simulink model "VIRTUAL_self_driving_stack_v2"  (R2025b)
settings: Solver=ode1  StartTime=0.0  StopTime=inf  FixedStep=Controller_Sample_Time  RelTol=1e-3  EnableMultiTasking=on
values from neighbouring files (symbols this model uses):
  angles_qcar2 = angles_new_qcar2(2: length (angles_new_qcar2), width (angles_new_qcar2)-5)    [Setup_QCar2_Params.m]
  cal_pos = [0, 0, 0]    [Setup_QCar2_Params.m]
  Controller_Sample_Time = 1/500    (= 0.002)    [Setup_QCar2_Params.m]
  CSI_Sample_Time = Controller_Sample_Time * ceil(0.033 / Controller_Sample_Time)    [Setup_QCar2_Params.m]
  dropoffXY = pathXY(dropoffPathIndex,:)    [example_sdcs_path.m]
  GyroKF_P0 = eye(2)    [Setup_QCar2_Params.m]
  GyroKF_Q = diag([0.01, 0.001])    [Setup_QCar2_Params.m]
  GyroKF_R = 0.01    [Setup_QCar2_Params.m]
  GyroKF_X0 = [0;0]    [Setup_QCar2_Params.m]
  ImageDisplay_Sample_Time = Controller_Sample_Time * 50    (= 0.1)    [Setup_QCar2_Params.m]
  Initialization_Time = 5    [Setup_QCar2_Params.m]
  LiDAR_Sample_Time = Controller_Sample_Time * ceil(1/15 / Controller_Sample_Time)    [Setup_QCar2_Params.m]
  N = size(roadmap.nodes,1)    [example_sdcs_path.m]
  path_x4 = path_x_custom    [Setup_QCar2_Params.m]
  path_y4 = path_y_custom    [Setup_QCar2_Params.m]
  pickupXY = pathXY(pickupPathIndex,:)    [example_sdcs_path.m]
  qcar2_lidar_to_body_rotation = -pi    (= -3.14159265359)    [Setup_QCar2_Params.m]
  qcar2_lidar_to_map_rotation = 2*pi/180    (= 0.0349065850399)    [Setup_QCar2_Params.m]
  qcar2_virtual_to_physical_lidar_rotation = 0    [Setup_QCar2_Params.m]
  QCarEKF_L = 0.256    [Setup_QCar2_Params.m]
  QCarEKF_P0 = eye(3)    [Setup_QCar2_Params.m]
  QCarEKF_Q = diag([0.00001, 0.00001, 0.00001])    [Setup_QCar2_Params.m]
  QCarEKF_R_combined = diag([0.1, 0.1, 0.01])    [Setup_QCar2_Params.m]
  QCarEKF_R_heading = diag(0.1)    [Setup_QCar2_Params.m]
  QcarKF_X0 = [0; 0; 0]    [Setup_QCar2_Params.m]
  range_qcar2 = distance_new_qcar2(2: length (distance_new_qcar2), width (distance_new_qcar2)-5)    [Setup_QCar2_Params.m]
  RealSense_Sample_Time = Controller_Sample_Time * ceil(0.033 / Controller_Sample_Time)    [Setup_QCar2_Params.m]
  steering_Kd = 0.1    [Setup_QCar2_Params.m]
  taxiHubXY = pathXY(taxiHubPathIndex,:)    [example_sdcs_path.m]
  x = roadmap.nodes(i,1)    [example_sdcs_path.m]
undefined symbols (not defined in the file or in its folder): AAAF5050, gcbh, height, HIL, JPEG, K12, left, MC, Point, qc_get_step_size, top, Video3D, video_display_show, width
libraries: quarc_library x76, simulink x17, simulink_extras x4, visiontextngfix x1
(part 4 of 4)

== system VIRTUAL_self_driving_stack_v2/Image Processing/ImageProcessingBlock/colorThresholdingHSV ==
  note: Generate the thresholded binary
  note: Transform RGB Image to an HSV one
  note: Color wheel
      | reference
      | for Hue_360
  note: HSV-Color Thresholding Module:
      |
      | This subsystem thresholds a given RGB image based on the desired colour and hue
      |
      | Inputs:
      | imageRGB (uint8) {0,255} : Input RGB Image to be thresholded
      | desiredHue (int) {-1}U{0,360} : Desired Hue to threshold around (provided in the 0-360 degree range, see the color wheel for hue selection)
      | Set the desired hue to -1 if you are interested in thresholding for white
      | [Sat_min, Val_min] (uint8) {0,255} : Minimum Saturation and Value thresholds
      | [Sat_max, Val_max] (uint8) {0,255} : Maximum Saturation and Value thresholds
      |
      | Outputs:
      | imageBinary (uint8) {0,255} : Binary Image (0 or 255 and no other value) representing the thresholding output
      |
      | Usage:
      | This module can be used when you are interested in thresholding for a certain hue regardless of the luminance. Compared to RGB thresholding which does not work well when the lighting conditions vary, HSV thresholding will correctly threshold for a hue (color) and allow you to specify a broad range of illuminance via the saturation and value thresholds. To broaden the range of hues accepted in the thresholding block, increase the Hue Threshold parameter.
  imageHSV : Inport
  desiredHue : Inport  Port=2
  "[Sat_min, Val_min]" : Inport  Port=3
  "[Sat_max, Val_max]" : Inport  Port=4
  Add3 : Sum
  Add4 : Sum  Inputs=-+
  Compare To Constant : simulink/Logic and Bit Operations/Compare To Constant  relop===  const=-1  OutDataTypeStr=boolean
  Constant : Constant  Value=0
  Constant1 : Constant  Value=255
  Display : Display
  Gain : Gain  Gain=255/360
  HSV Color Thresholding : quarc_library/Image Processing/Generic/Image Compare  output_type=Combined (one HxW output)  source=External input ports  r_comparison=min <= pixel and pixel <= max with wrapping  r_minimum=30  r_maximum=70  g_comparison=min <= pixel and pixel <= max  g_minimum=60  g_maximum=100  b_comparison=min <= pixel and pixel <= max  b_minimum=40  b_maximum=80
      settings: SourceProductName=QUARC Targets
  Hue Threshold : Constant  Value=20
  Mux1 : Mux  Inputs=2
  Mux2 : Mux  Inputs=2
  Switch : Switch  Criteria=u2 > Threshold  SaturateOnIntegerOverflow=off  InputSameDT=off
  Switch1 : Switch  Criteria=u2 > Threshold  SaturateOnIntegerOverflow=off  InputSameDT=off
  imageBinary : Outport  VectorParamsAs1DForOutWhenUnconnected=off
  wires:
  Hue Threshold/1 -> Add3/1, Add4/1
  imageHSV/1 -> HSV Color Thresholding/1
  desiredHue/1 -> Compare To Constant/1, Display/1, Gain/1
  Gain/1 -> Add4/2, Add3/2
  Constant1/1 -> Switch1/1
  "[Sat_max, Val_max]"/1 -> Mux1/2
  Add3/1 -> Switch1/3
  Switch/1 -> Mux2/1
  Compare To Constant/1 -> Switch/2, Switch1/2
  Constant/1 -> Switch/1
  Switch1/1 -> Mux1/1
  Mux1/1 -> HSV Color Thresholding/3
  Add4/1 -> Switch/3
  "[Sat_min, Val_min]"/1 -> Mux2/2
  Mux2/1 -> HSV Color Thresholding/2
  HSV Color Thresholding/1 -> imageBinary/1

== system VIRTUAL_self_driving_stack_v2/Image Processing/findStopSignDistance/Depth Image (m) ==
  In1 : Inport
  Channel : quarc_library/Signal Routing/Channel  channel=5  buffer_size=1
  Image Compress : quarc_library/Image Processing/Generic/Image Compress  algorithm=JPEG  source=Internal dialog parameter  quality=quality  output_dim=-1
  Video Display : quarc_library/Multimedia/Video Display  Tag=VIRTUAL_self_driving_stack_v2/Image Processing/findStopSignDistance/Depth Image (m)/Video Display  sample_time=sample_time  use_hardware=on
  wires:
  Image Compress/1 -> Channel/1
  In1/1 -> Image Compress/1
  Channel/1 -> Video Display/1

== system VIRTUAL_self_driving_stack_v2/lidarLocalization/rising edge latch/Latch Input ==
  Input : Inport
  Trigger : TriggerPort  VariantControl=(inherit)
  Constant : Constant
  Latch : Outport  VectorParamsAs1DForOutWhenUnconnected=off
  Executed : Outport  Port=2  VectorParamsAs1DForOutWhenUnconnected=off
  wires:
  Constant/1 -> Executed/1
  Input/1 -> Latch/1

== system VIRTUAL_self_driving_stack_v2/stateEstimation/Fusion Comparison & Kalman Estimator/Angle mod1 ==
  Angle : Inport
  Bias : Bias  Bias=180  SaturateOnIntegerOverflow=off
  Bias1 : Bias  Bias=-180  SaturateOnIntegerOverflow=off
  Constant1 : Constant  Value=360
  Mod : Math  Operator=mod
  Mod_Angle : Outport
  wires:
  Angle/1 -> Bias/1
  Bias1/1 -> Mod_Angle/1
  Bias/1 -> Mod/1
  Constant1/1 -> Mod/2
  Mod/1 -> Bias1/1

== system VIRTUAL_self_driving_stack_v2/steeringCommander/Steering Based on LiDAR/If Action Subsystem ==
  aoa [1] (rad) : Inport
  Action Port : ActionPort  ActionPortLabel=if(u1 < -pi)
  Bias : Bias  Bias=2*pi  SaturateOnIntegerOverflow=off
  steering [1] (rad) : Outport
  wires:
  aoa [1] (rad)/1 -> Bias/1
  Bias/1 -> steering [1] (rad)/1

== system VIRTUAL_self_driving_stack_v2/steeringCommander/Steering Based on LiDAR/If Action Subsystem1 ==
  aoa [1] (rad) : Inport
  Action Port : ActionPort  ActionPortLabel=elseif(u1 > pi)
  Bias : Bias  Bias=-2*pi  SaturateOnIntegerOverflow=off
  steering [1] (rad) : Outport
  wires:
  Bias/1 -> steering [1] (rad)/1
  aoa [1] (rad)/1 -> Bias/1

== system VIRTUAL_self_driving_stack_v2/steeringCommander/Steering Based on LiDAR/If Action Subsystem2 ==
  aoa [1] (rad) : Inport
  Action Port : ActionPort  ActionPortLabel=else
  Bias : Bias  SaturateOnIntegerOverflow=off
  steering [1] (rad) : Outport
  wires:
  aoa [1] (rad)/1 -> Bias/1
  Bias/1 -> steering [1] (rad)/1

== system VIRTUAL_self_driving_stack_v2/Image Processing/ImageProcessingBlock/DetectTrafficLight/Binary showing Green ==
  In1 : Inport
  Channel : quarc_library/Signal Routing/Channel  channel=2  buffer_size=1
  Image Compress : quarc_library/Image Processing/Generic/Image Compress  algorithm=JPEG  source=Internal dialog parameter  quality=quality  output_dim=-1
  Video Display : quarc_library/Multimedia/Video Display  Tag=VIRTUAL_self_driving_stack_v2/Image Processing/ImageProcessingBlock/DetectTrafficLight/Binary showing Green/Video Display  sample_time=sample_time  use_hardware=on
  wires:
  Image Compress/1 -> Channel/1
  In1/1 -> Image Compress/1
  Channel/1 -> Video Display/1

== system VIRTUAL_self_driving_stack_v2/Image Processing/ImageProcessingBlock/DetectTrafficLight/Binary showing Red ==
  In1 : Inport
  Channel : quarc_library/Signal Routing/Channel  channel=3  buffer_size=1
  Image Compress : quarc_library/Image Processing/Generic/Image Compress  algorithm=JPEG  source=Internal dialog parameter  quality=quality  output_dim=-1
  Video Display : quarc_library/Multimedia/Video Display  Tag=VIRTUAL_self_driving_stack_v2/Image Processing/ImageProcessingBlock/DetectTrafficLight/Binary showing Red/Video Display  sample_time=sample_time  use_hardware=on
  wires:
  Image Compress/1 -> Channel/1
  In1/1 -> Image Compress/1
  Channel/1 -> Video Display/1

== system VIRTUAL_self_driving_stack_v2/Image Processing/ImageProcessingBlock/DetectTrafficLight/colorThresholdingGreen ==
  note: Generate the thresholded binary
  note: Transform RGB Image to an HSV one
  note: Color wheel
      | reference
      | for Hue_360
  note: HSV-Color Thresholding Module:
      |
      | This subsystem thresholds a given RGB image based on the desired colour and hue
      |
      | Inputs:
      | imageRGB (uint8) {0,255} : Input RGB Image to be thresholded
      | desiredHue (int) {-1}U{0,360} : Desired Hue to threshold around (provided in the 0-360 degree range, see the color wheel for hue selection)
      | Set the desired hue to -1 if you are interested in thresholding for white
      | [Sat_min, Val_min] (uint8) {0,255} : Minimum Saturation and Value thresholds
      | [Sat_max, Val_max] (uint8) {0,255} : Maximum Saturation and Value thresholds
      |
      | Outputs:
      | imageBinary (uint8) {0,255} : Binary Image (0 or 255 and no other value) representing the thresholding output
      |
      | Usage:
      | This module can be used when you are interested in thresholding for a certain hue regardless of the luminance. Compared to RGB thresholding which does not work well when the lighting conditions vary, HSV thresholding will correctly threshold for a hue (color) and allow you to specify a broad range of illuminance via the saturation and value thresholds. To broaden the range of hues accepted in the thresholding block, increase the Hue Threshold parameter.
  imageHSV : Inport
  desiredHue : Inport  Port=2
  "[Sat_min, Val_min]" : Inport  Port=3
  "[Sat_max, Val_max]" : Inport  Port=4
  Add3 : Sum
  Add4 : Sum  Inputs=-+
  Compare To Constant : simulink/Logic and Bit Operations/Compare To Constant  relop===  const=-1  OutDataTypeStr=boolean
  Constant : Constant  Value=0
  Constant1 : Constant  Value=255
  Display : Display
  Gain : Gain  Gain=255/360
  HSV Color Thresholding : quarc_library/Image Processing/Generic/Image Compare  output_type=Combined (one HxW output)  source=External input ports  r_comparison=min <= pixel and pixel <= max with wrapping  r_minimum=30  r_maximum=70  g_comparison=min <= pixel and pixel <= max  g_minimum=60  g_maximum=100  b_comparison=min <= pixel and pixel <= max  b_minimum=40  b_maximum=80
      settings: SourceProductName=QUARC Targets
  Hue Threshold : Constant  Value=20
  Mux1 : Mux  Inputs=2
  Mux2 : Mux  Inputs=2
  Switch : Switch  Criteria=u2 > Threshold  SaturateOnIntegerOverflow=off  InputSameDT=off
  Switch1 : Switch  Criteria=u2 > Threshold  SaturateOnIntegerOverflow=off  InputSameDT=off
  imageBinary : Outport  VectorParamsAs1DForOutWhenUnconnected=off
  wires:
  Hue Threshold/1 -> Add3/1, Add4/1
  imageHSV/1 -> HSV Color Thresholding/1
  desiredHue/1 -> Compare To Constant/1, Display/1, Gain/1
  Gain/1 -> Add4/2, Add3/2
  Constant1/1 -> Switch1/1
  "[Sat_max, Val_max]"/1 -> Mux1/2
  Add3/1 -> Switch1/3
  Switch/1 -> Mux2/1
  Compare To Constant/1 -> Switch/2, Switch1/2
  Constant/1 -> Switch/1
  Switch1/1 -> Mux1/1
  Mux1/1 -> HSV Color Thresholding/3
  Add4/1 -> Switch/3
  "[Sat_min, Val_min]"/1 -> Mux2/2
  Mux2/1 -> HSV Color Thresholding/2
  HSV Color Thresholding/1 -> imageBinary/1

== system VIRTUAL_self_driving_stack_v2/Image Processing/ImageProcessingBlock/DetectTrafficLight/colorThresholdingRed ==
  note: Generate the thresholded binary
  note: Transform RGB Image to an HSV one
  note: Color wheel
      | reference
      | for Hue_360
  note: HSV-Color Thresholding Module:
      |
      | This subsystem thresholds a given RGB image based on the desired colour and hue
      |
      | Inputs:
      | imageRGB (uint8) {0,255} : Input RGB Image to be thresholded
      | desiredHue (int) {-1}U{0,360} : Desired Hue to threshold around (provided in the 0-360 degree range, see the color wheel for hue selection)
      | Set the desired hue to -1 if you are interested in thresholding for white
      | [Sat_min, Val_min] (uint8) {0,255} : Minimum Saturation and Value thresholds
      | [Sat_max, Val_max] (uint8) {0,255} : Maximum Saturation and Value thresholds
      |
      | Outputs:
      | imageBinary (uint8) {0,255} : Binary Image (0 or 255 and no other value) representing the thresholding output
      |
      | Usage:
      | This module can be used when you are interested in thresholding for a certain hue regardless of the luminance. Compared to RGB thresholding which does not work well when the lighting conditions vary, HSV thresholding will correctly threshold for a hue (color) and allow you to specify a broad range of illuminance via the saturation and value thresholds. To broaden the range of hues accepted in the thresholding block, increase the Hue Threshold parameter.
  imageHSV : Inport
  desiredHue : Inport  Port=2
  "[Sat_min, Val_min]" : Inport  Port=3
  "[Sat_max, Val_max]" : Inport  Port=4
  Add3 : Sum
  Add4 : Sum  Inputs=-+
  Compare To Constant : simulink/Logic and Bit Operations/Compare To Constant  relop===  const=-1  OutDataTypeStr=boolean
  Constant : Constant  Value=0
  Constant1 : Constant  Value=255
  Display : Display
  Gain : Gain  Gain=255/360
  HSV Color Thresholding : quarc_library/Image Processing/Generic/Image Compare  output_type=Combined (one HxW output)  source=External input ports  r_comparison=min <= pixel and pixel <= max with wrapping  r_minimum=30  r_maximum=70  g_comparison=min <= pixel and pixel <= max  g_minimum=60  g_maximum=100  b_comparison=min <= pixel and pixel <= max  b_minimum=40  b_maximum=80
      settings: SourceProductName=QUARC Targets
  Hue Threshold : Constant  Value=20
  Mux1 : Mux  Inputs=2
  Mux2 : Mux  Inputs=2
  Switch : Switch  Criteria=u2 > Threshold  SaturateOnIntegerOverflow=off  InputSameDT=off
  Switch1 : Switch  Criteria=u2 > Threshold  SaturateOnIntegerOverflow=off  InputSameDT=off
  imageBinary : Outport  VectorParamsAs1DForOutWhenUnconnected=off
  wires:
  Hue Threshold/1 -> Add3/1, Add4/1
  imageHSV/1 -> HSV Color Thresholding/1
  desiredHue/1 -> Compare To Constant/1, Display/1, Gain/1
  Gain/1 -> Add4/2, Add3/2
  Constant1/1 -> Switch1/1
  "[Sat_max, Val_max]"/1 -> Mux1/2
  Add3/1 -> Switch1/3
  Switch/1 -> Mux2/1
  Compare To Constant/1 -> Switch/2, Switch1/2
  Constant/1 -> Switch/1
  Switch1/1 -> Mux1/1
  Mux1/1 -> HSV Color Thresholding/3
  Add4/1 -> Switch/3
  "[Sat_min, Val_min]"/1 -> Mux2/2
  Mux2/1 -> HSV Color Thresholding/2
  HSV Color Thresholding/1 -> imageBinary/1

== matlab function VIRTUAL_self_driving_stack_v2/stateEstimation/Sensor Fusion - Complementary Filter/MATLAB Function ==
  data: car_speed input; correction_weight output; slope input; min_weight input
function correction_weight = weighting(car_speed, slope, min_weight)
correction_weight = 1 - 1*slope*car_speed;
if correction_weight < min_weight
    correction_weight = min_weight;
end
end

== matlab function VIRTUAL_self_driving_stack_v2/Image Processing/ImageProcessingBlock/DetectTrafficLight/MATLAB Function ==
  data: imageHSV input; meanV output; imageBinary input
function meanV = computeMeanV(imageHSV, imageBinary)
% imageHSV: HxWx3 uint8
% imageBinary: HxW uint8, values 0 or 255

V = imageHSV(:,:,3);

mask = imageBinary > 0;

vals = V(mask);

if isempty(vals)
    meanV = 0;
else
    meanV = mean(double(vals));
end

== matlab function VIRTUAL_self_driving_stack_v2/Image Processing/ImageProcessingBlock/DetectTrafficLight/MATLAB Function1 ==
  data: imageHSV input; meanV output; imageBinary input
function meanV = computeMeanV(imageHSV, imageBinary)
%#codegen
V = imageHSV(:,:,3);
mask = imageBinary > 0;
vals = V(mask);

if isempty(vals)
    meanV = 0;
else
    % If we find even ONE red pixel, return 255 to force the stop
    % This helps us check if the HSV mask is working
    meanV = 255; 
end

== matlab function VIRTUAL_self_driving_stack_v2/Image Processing/ImageProcessingBlock/MATLAB Function2 ==
  data: circularity output; box input; area input; extent output
function [circularity,extent] = detect_sign_from_area(box, area)

%#codegen
% sign_type:
% 0 = unknown
% 1 = yield
% 2 = stop


% Extract box
min_row = double(box(1));
min_col = double(box(2));
max_row = double(box(3));
max_col = double(box(4));

% Compute dimensions
height = max_row - min_row;
width  = max_col - min_col;

% Approximate perimeter
perimeter = 2 * (height + width);

% Circularity
circularity = 4 * pi * double(area) / (perimeter^2);

% Extent (how filled the box is)
box_area = height * width;
extent = double(area) / double(box_area);

% ---------- CLASSIFICATION ----------

% STOP (octagon)
% if circularity > 0.7 && extent > 0.6
%     sign_type = uint8(2);
% 
% % YIELD (triangle)
% elseif circularity > 0.45 && circularity < 0.7 && extent < 0.7
%     sign_type = uint8(1);
% 
% else
%     sign_type = uint8(0);
% end

end

== matlab function VIRTUAL_self_driving_stack_v2/speedController/realsenseObstacleDetectionSpeedAdjust/MATLAB Function ==
  data: obstacle_distance input; speed_cmd output; stop_distance input; nominal_tracking_distance input; nominal_speed input
function speed_cmd = adaptive_cruise_control(obstacle_distance, stop_distance, nominal_tracking_distance, nominal_speed)

speed_cmd = nominal_speed;

if obstacle_distance < stop_distance
    speed_cmd = sat(nominal_speed,0,-1);
    
elseif obstacle_distance < nominal_tracking_distance
    speed_cmd = nominal_speed/(nominal_tracking_distance-stop_distance)*obstacle_distance...
        - nominal_speed/(nominal_tracking_distance-stop_distance)*stop_distance;
    
end

function output = sat (input, max,min)
if input > max
    output = max;
elseif input < min
    output = min;
else
    output = input;
end

== matlab function VIRTUAL_self_driving_stack_v2/speedController/MATLAB Function1 ==
  data: speedIn input; dt input; reset input; speedOut output
function speedOut = startupRamp(speedIn, dt, reset)
%#codegen
% speedIn: The desired speed (e.g., 0.5) coming from your logic
% dt: Simulation sample time (e.g., 0.002)
% speedOut: The ramped speed sent to the controller

    persistent totalTime
    
    % 1. Initialize the timer
    if isempty(totalTime)
        totalTime = 0.0;
    end
    
    % 2. Reset if simulation restarts
    if reset > 0.5
        totalTime = 0.0;
    end

    % 3. Increment time
    totalTime = totalTime + dt;

    % 4. The 10-Second Progressive Logic
    if totalTime <= 10.0
        % Calculate factor: 0 at t=0, reaching 1.0 at t=10
        alpha = totalTime / 10.0;
        speedOut = speedIn * alpha;
    else
        % AFTER 10 SECONDS:
        % The ramp is "dead." Pass the signal through perfectly.
        % This ensures traffic light changes (0 to 0.5) are INSTANT.
        speedOut = speedIn;
    end
end

== matlab function VIRTUAL_self_driving_stack_v2/obstacleDetection/obstacleDetection Markham March 22/Draw Lines Module ==
  data: img_in input; img_out output; pts input; color input
function img_out = drawLines(img_in, pts, color)

% Draw lines connecting the points using the provided color

% Inputs:
% u         : Input RGB Image (size = m by n)
% pts       : p x-y pairs of points (px) where markers are to be drawn
% color     : 1x3 matrix of RGB color values for each marker

% Outputs:
% y         : Output RGB Image with the markers drawn in (size = m by n)

%% Initialization
if size(img_in, 3) == 3
    img_out = img_in;
elseif size(img_in, 3) == 1
    img_out = cat(3, img_in, img_in, img_in);
end

[p, ~] = size(pts); % determine the number of points

%% Draw the lines
    for i = 1:p-1
        % determine the max(rows_difference, col_difference) between two
        % points
        itr = max(abs(pts(i,1) - pts(i+1,1)), abs(pts(i,2) - pts(i+1,2)));
        
        % generate linear spaces of row and col values between the pts
        row_vec = round(linspace(pts(i,1), pts(i+1,1), itr));
        col_vec = round(linspace(pts(i,2), pts(i+1,2), itr));
        
        % iterate through the values and shade them right

        for j = 1:itr
            img_out(row_vec(j), col_vec(j),1) = color(1);
            img_out(row_vec(j), col_vec(j),2) = color(2);
            img_out(row_vec(j), col_vec(j),3) = color(3);
        end
    end
end

== matlab function VIRTUAL_self_driving_stack_v2/obstacleDetection/obstacleDetection Markham March 22/Steering based image subselector ==
  data: pts output; depth input; distance output; steering input; minDistance input; maxDistance input; width input; height input; vertCenter input; maxSteering input; reduction input; maxSteeringWidth input
function [pts, distance] = estimateDepthInRegion(depth, steering, minDistance, maxDistance, width, height, vertCenter, maxSteering, reduction, maxSteeringWidth)
% Input: 640 x 360
[ROW, COL] = size(depth);
mark = COL/2 - (steering*(COL/2 - width/2)/maxSteering);
applied_width = max(width - abs(steering/maxSteeringWidth)*reduction*width, 60);
left_w = max(mark+1-(applied_width/2), 0); % pick the left end, but never let it get negative
right_w = min(left_w + applied_width, COL); % pick the right end, but never past the image width
upper_h = max(ROW*vertCenter-height/2+1, 0); % pick the upper end, but never let it get negative
lower_h = min(ROW*vertCenter+height/2, ROW); % pick the lower end, but never let it go past the image height
depth(:,1:40) = maxDistance; %this is to remove artifacts in the camera's left section
region = double(depth(upper_h:lower_h, left_w:right_w)); 
pts = [upper_h, left_w; upper_h, right_w; lower_h, right_w; lower_h, left_w; upper_h, left_w];
u_flat = reshape(region, 1, []);

temp = maxDistance*ones(1, length(u_flat));

for i = 1:length(u_flat)
    if (u_flat(i) >= minDistance) && (u_flat(i) <= maxDistance)
        temp(i) = u_flat(i);
    end
end

% u_flat(u_flat < minDistance) = [];
% u_flat(u_flat > maxDistance) = [];
% distance = mean(mean(u_flat));
distance = min(temp(:));

== matlab function VIRTUAL_self_driving_stack_v2/stateEstimation/Gyro KF + EKF/Heading Kalman Filter ==
  settings: updateMethod=DISCRETE
  data: thd_gyro input; th_gps input; newGPSData input; GyroKF_Q parameter; GyroKF_R parameter; GyroKF_X0 parameter; GyroKF_P0 parameter; th_hat output; gyro_bias output; Controller_Sample_Time parameter
function [th_hat, gyro_bias] = GyroKF(thd_gyro, th_gps, newGPSData, GyroKF_Q, GyroKF_R, GyroKF_X0, GyroKF_P0, Controller_Sample_Time)

    persistent X_hat P I A B C
    if isempty(X_hat)
        % State and Covarience estimates
        X_hat = GyroKF_X0;
        P = GyroKF_P0;

        % Statespace model matrices
        I = eye(2);
        A = I + Controller_Sample_Time*[0, -1;
                                   0, 0];
        B = Controller_Sample_Time*[1;
                               0];
        C = [1, 0];
    end

    % Prediction
    X_hat = A*X_hat + B*thd_gyro;
    P = A*P*A' + GyroKF_Q;

    % Correction 
    if newGPSData
        P_times_CTransposed = P*C';
        S = C*P_times_CTransposed + GyroKF_R;
        K = P_times_CTransposed / S;

        z = wrapToPi(th_gps - C*X_hat);

        X_hat = X_hat + K*z;
        X_hat(1) = wrapToPi(X_hat(1));

        P = (I - K*C) * P;
    end
    
    th_hat = X_hat(1);
    gyro_bias = X_hat(2);
end

== matlab function VIRTUAL_self_driving_stack_v2/stateEstimation/Gyro KF + EKF/QCar EKF ==
  settings: updateMethod=DISCRETE
  data: speed input; delta input; x_gps input; Xhat output; y_gps input; th_hat input; newGPSData input; Controller_Sample_Time parameter; QCarEKF_P0 parameter; QcarKF_X0 parameter; QCarEKF_R_heading parameter; QCarEKF_Q parameter; QCarEKF_L parameter; QCarEKF_R_combined parameter
function Xhat  = QCarEKF(speed, delta, x_gps, y_gps, th_hat, newGPSData, Controller_Sample_Time, QCarEKF_P0, QcarKF_X0, QCarEKF_R_heading, QCarEKF_Q, QCarEKF_L, QCarEKF_R_combined)




    persistent X_hat P I C_heading C_combined
    if isempty(X_hat)
        % State and Covarience estimates
        X_hat = QcarKF_X0;
        P = QCarEKF_P0;

        % Statespace model matrices
        I = eye(3);
        
        C_heading = [0, 0, 1];
        C_combined = eye(3);
    end
    
    dt = Controller_Sample_Time;
    x = X_hat(1);
    y = X_hat(2);
    th = X_hat(3);
    
    % Prediction:
    F = [1, 0, -dt*speed*sin(th);
         0, 1,  dt*speed*cos(th);
         0, 0,             1];
    P = F*P*F' + QCarEKF_Q;
    
    X_hat = X_hat + dt*speed * [cos(th);
                            sin(th);
                            tan(delta) / QCarEKF_L];
                         
    
    % Correction
    if newGPSData
        y = [x_gps; y_gps; th_hat];
        C = C_combined;
        R = QCarEKF_R_combined;
        
    else
        y = th_hat;
        C = C_heading;
        R = QCarEKF_R_heading;
    end

    P_times_CTransposed = P*C';
    S = C*P_times_CTransposed + R;
    K = P_times_CTransposed / S;

    z = y - C*X_hat;
    if newGPSData
        z(3) = wrapToPi(z(3));
    else
        z = wrapToPi(z);
    end

    X_hat = X_hat + K*z;
    X_hat(3) = wrapToPi(X_hat(3));

    P = (I - K*C) * P;
    
    Xhat = X_hat;
end

== matlab function VIRTUAL_self_driving_stack_v2/lidarLocalization/Match Scans/MATLAB Function ==
  data: new_range output size=SPR_qcar2 [..SPR_qcar2]; range input [1..SPR_qcar2]; angles input [1..SPR_qcar2]; new_angles output size=SPR_qcar2 [..SPR_qcar2]
function [new_range, new_angles]  = clean_zero_readings(range, angles)
range_indicies = find (range == 0);
range(range_indicies) = [];
angles(range_indicies) = [];
new_range = range;
new_angles = angles;
end

== matlab function VIRTUAL_self_driving_stack_v2/speedController/Subsystem/MATLAB Function ==
  settings: updateMethod=DISCRETE
  data: throttleIn input; throttleOut output; xCurrent input; yCurrent input; hubX input; hubY input; pickupX input; pickupY input; dropoffX input; dropoffY input; stopSign input; greenTraffic input; redTraffic input; distToSign input; dt input; reset input; rgb output; isStopped output; resumeAlpha output; stageOut output; missionDone output; leds output
function [throttleOut, rgb, isStopped, resumeAlpha, stageOut, missionDone, leds] = taxiMissionThrottleGate( ...
    throttleIn, xCurrent, yCurrent, hubX, hubY, pickupX, pickupY, dropoffX, dropoffY, ...
    stopSign, greenTraffic, redTraffic, distToSign, dt, reset)
%#codegen

    % --- Persistent Variables ---
    persistent totalTime
    persistent stage stopActive stopTimer targetLatched done
    persistent resumeActive resumeTimer
    persistent steeringHoldActive steeringHoldTimer
    persistent trafficStopActive trafficTimer signProcessed
    
    % --- 1. INITIALIZATION ---
    if isempty(totalTime);          totalTime          = 0.0;      end
    if isempty(stage);              stage              = int32(0); end
    if isempty(stopActive);         stopActive         = false;    end
    if isempty(stopTimer);          stopTimer          = 0.0;      end
    if isempty(targetLatched);      targetLatched      = false;    end
    if isempty(done);               done               = false;    end
    if isempty(resumeActive);       resumeActive       = false;    end
    if isempty(resumeTimer);        resumeTimer        = 0.0;      end
    if isempty(steeringHoldActive); steeringHoldActive = false;    end
    if isempty(steeringHoldTimer);  steeringHoldTimer  = 0.0;      end
    if isempty(trafficStopActive);  trafficStopActive  = false;    end
    if isempty(trafficTimer);       trafficTimer       = 0.0;      end
    if isempty(signProcessed);      signProcessed      = false;    end

    % --- 2. DEFAULT OUTPUTS ---
    isStopped   = 0.0;
    resumeAlpha = 1.0;
    throttleOut = throttleIn;
    rgb         = [1.0 0.0 1.0];   % Default Magenta
    missionDone = 0.0;
    stageOut    = double(stage);
    totalTime   = totalTime + dt;

    % 16 bool leds — column vector to match HIL Write port [16x1]
    % leds(1-4)    = brake lights  (LEDs 11-14)
    % leds(6-7)    = rear signals  (LEDs 16-17)
    % leds(8,9,11,12) = headlights (LEDs 18,19,21,22)
    leds = [false false false false false false false false ...
            false false false false false false false false]';

    % --- Constants ---
    threshold            = 0.27;
    stopDuration         = 3.0;
    steeringHoldDuration = 2.1;
    resumeDuration       = 4.0;
    trafficWaitDuration  = 2.0;
    redLightBuffer       = 1.5;
    distThreshold        = 1.1;

    % --- 3. RESET LOGIC ---
    if reset ~= 0
        totalTime = 0.0; stage = int32(0); stopActive = false; stopTimer = 0.0;
        targetLatched = false; done = false; resumeActive = false; resumeTimer = 0.0;
        steeringHoldActive = false; steeringHoldTimer = 0.0;
        trafficStopActive = false; trafficTimer = 0.0; signProcessed = false;
        return;
    end

    % --- 4. TRAFFIC & STOP SIGN LOGIC ---
    if greenTraffic > 0.5
        trafficStopActive = false;
        trafficTimer      = 0.0;
    elseif redTraffic > 0.5
        trafficStopActive = true;
        trafficTimer      = redLightBuffer;
    elseif (stopSign > 0.5) && (~signProcessed) && ...
           (distToSign < distThreshold) && (distToSign > 0.1)
        trafficStopActive = true;
        trafficTimer      = trafficWaitDuration;
        signProcessed     = true;
    elseif trafficStopActive
        trafficTimer = trafficTimer - dt;
        if trafficTimer <= 0.0 && redTraffic < 0.5
            trafficStopActive = false;
        end
    end
    if stopSign < 0.5
        signProcessed = false;
    end

    % --- 5. MISSION TARGET LOGIC ---
    if stage == 0
        targetX = pickupX;  targetY = pickupY;
    elseif stage == 1
        targetX = dropoffX; targetY = dropoffY;
    else
        targetX = hubX;     targetY = hubY;
    end

    dist = sqrt((xCurrent - targetX)^2 + (yCurrent - targetY)^2);

    if (~stopActive) && (~steeringHoldActive) && (~resumeActive) && ...
       (~done) && (dist <= threshold) && (~targetLatched)
        targetLatched = true;
        if stage == 0 || stage == 1
            stopActive = true;
            stopTimer  = stopDuration;
        else
            done = true;
        end
    end

    % --- 6. TIMERS ---
    if stopActive
        stopTimer = stopTimer - dt;
        if stopTimer <= 0.0
            stopActive = false;
            if stage == 0;     stage = int32(1);
            elseif stage == 1; stage = int32(2); end
            if ~done
                steeringHoldActive = true;
                steeringHoldTimer  = steeringHoldDuration;
            end
        end
    end

    if steeringHoldActive
        steeringHoldTimer = steeringHoldTimer - dt;
        if steeringHoldTimer <= 0.0
            steeringHoldActive = false;
            if ~done
                resumeActive = true;
                resumeTimer  = resumeDuration;
            end
        end
    end

    if resumeActive
        resumeTimer = resumeTimer - dt;
        if resumeTimer <= 0.0
            resumeActive = false;
        end
    end

    if dist > threshold
        targetLatched = false;
    end

    % --- 7. ACTUATORS & LEDs ---
    startupAlpha = min(1.0, totalTime / 10.0);

    if stopActive || steeringHoldActive || trafficStopActive
        % ANY STOP → brake lights ON
        isStopped   = 1.0;
        resumeAlpha = 0.0;
        throttleOut = 0.0;
        leds(1) = true;   % LED 11: left outside brake
        leds(2) = true;   % LED 12: left inside brake
        leds(3) = true;   % LED 13: right inside brake
        leds(4) = true;   % LED 14: right outside brake

    elseif resumeActive
        % RESUMING → headlights + rear signals
        isStopped   = 0.0;
        resumeAlpha = max(0.0, min(1.0, 1.0 - (resumeTimer / resumeDuration)));
        throttleOut = throttleIn * (resumeAlpha * resumeAlpha * resumeAlpha) * startupAlpha;
        leds(6)  = true;   % LED 16: left rear signal
        leds(7)  = true;   % LED 17: right rear signal
        leds(8)  = true;   % LED 18: left outside headlight
        leds(9)  = true;   % LED 19: left middle headlight
        leds(11) = true;   % LED 21: right inside headlight
        leds(12) = true;   % LED 22: right middle headlight

    else
        % NORMAL DRIVE → headlights only
        isStopped   = 0.0;
        resumeAlpha = 1.0;
        throttleOut = throttleIn * startupAlpha;
        if done; throttleOut = 0.0; end
        leds(8)  = true;   % LED 18: left outside headlight
        leds(9)  = true;   % LED 19: left middle headlight
        leds(11) = true;   % LED 21: right inside headlight
        leds(12) = true;   % LED 22: right middle headlight
    end

    % --- 8. RGB COLOR ---
    if done
        rgb = [1.0 0.0 1.0];       % Hub reached: Magenta

    elseif stage == 0
        rgb = [0.0 1.0 0.0];       % Navigating to pickup: Green

    elseif stage == 1
        rgb = [0.0 0.0 1.0];       % Carrying passenger: Blue

    elseif stage == 2
        rgb = [1.0 0.5 0.0];       % After dropoff: Orange
    end

    % Startup override — stay Magenta for first 10 seconds while
    % lidar initialises and system arms, then switch to Green
    if totalTime < 5.0 && stage == 0
        rgb = [1.0 0.0 1.0];       % Startup: Magenta
    end

    stageOut    = double(stage);
    missionDone = double(done);
end

== matlab function VIRTUAL_self_driving_stack_v2/pathPlanner/Path 4  Look Ahead Generator/Windowed Closest Point Locator *Feedback the location1 ==
  settings: updateMethod=DISCRETE
  data: x input; location output; y input; x_array input; y_array input; window input; global_search input; distance output; previous_location input; freezeTracking input
function [location,distance] = find_closest_window_point( ...
    x, y, x_array, y_array, window, global_search, previous_location, freezeTracking)
%#codegen

    persistent frozen_location prev_freeze

    distance = 1e6;
    location = previous_location;
    array_length = length(x_array);

    if isempty(frozen_location)
        frozen_location = previous_location;
    end
    if isempty(prev_freeze)
        prev_freeze = false;
    end

    % Safety clamp
    if previous_location < 1
        previous_location = 1;
    elseif previous_location > array_length
        previous_location = array_length;
    end

    freezeNow = (freezeTracking ~= 0);

    % ------------------------------------------------------------
    % On rising edge of freeze, latch the current valid location
    % ------------------------------------------------------------
    if freezeNow && (~prev_freeze)
        frozen_location = previous_location;
    end

    % ------------------------------------------------------------
    % If frozen, do not update location
    % ------------------------------------------------------------
    if freezeNow
        location = frozen_location;

        % safety clamp
        if location < 1
            location = 1;
        elseif location > array_length
            location = array_length;
        end

        dx = x - x_array(location);
        dy = y - y_array(location);
        distance = sqrt(dx*dx + dy*dy);

        prev_freeze = freezeNow;
        return;
    end

    % ------------------------------------------------------------
    % Normal search
    % ------------------------------------------------------------
    if (global_search == 1)

        % Search whole array at startup
        for i = 1:array_length
            d = (x - x_array(i))^2 + (y - y_array(i))^2;
            if d < distance
                distance = d;
                location = i;
            end
        end

    else

        % Forward-biased local search
        back_tolerance = 2;

        start_idx = previous_location - back_tolerance;
        end_idx = previous_location + window;

        if start_idx < 1
            start_idx = 1;
        end
        if end_idx > array_length
            end_idx = array_length;
        end

        for i = start_idx:end_idx
            d = (x - x_array(i))^2 + (y - y_array(i))^2;
            if d < distance
                distance = d;
                location = i;
            end
        end

        % Do not allow large backward jumps
        if location < previous_location - back_tolerance
            location = previous_location;
        end
    end

    distance = sqrt(distance);

    % Update stored frozen location when tracking is active
    frozen_location = location;
    prev_freeze = freezeNow;
end

== matlab function VIRTUAL_self_driving_stack_v2/steeringCommander/MATLAB Function ==
  data: isStopped input; dt input; holdZero output; releaseAlpha output; speedScale output
function [holdZero, releaseAlpha, speedScale] = holdAndReleaseSteering(isStopped, dt)
%#codegen
persistent releaseTimer releaseActive everStopped
if isempty(releaseTimer);  releaseTimer  = 0.0;   end
if isempty(releaseActive); releaseActive = false;  end
if isempty(everStopped);   everStopped   = false;  end

releaseDuration = 2.0;

% ── Stopped (Threshold check for noise) ──────────────────────────────────
if isStopped > 0.5 
    releaseTimer  = 0.0;
    releaseActive = false;
    everStopped   = true;   
    holdZero      = true;
    releaseAlpha  = 0.0;
    speedScale    = 0.0;
    return;
end

% ── Normal Drive (Pre-stop) ─────────────────────────────────────────────
if ~everStopped
    holdZero     = false;
    releaseAlpha = 1.0;
    speedScale   = 1.0;
    return;
end

% ── Trigger Release Phase ────────────────────────────────────────────────
if ~releaseActive
    releaseActive = true;
    releaseTimer  = releaseDuration;
end

if releaseActive
    releaseTimer = releaseTimer - dt;
    
    if releaseTimer <= 0.0
        releaseTimer  = 0.0;
        releaseActive = false;
        everStopped   = false;   
        holdZero      = false;
        releaseAlpha  = 1.0;
        speedScale    = 1.0;
        return;
    end
    
    % Calculate normalized progress (0 to 1)
    releaseAlpha = 1.0 - (releaseTimer / releaseDuration);
    
    % Modified Speed Scaling: Keeps speed very low (15%) initially 
    % to give the steering time to "bite" before accelerating.
    speedScale = 0.15 + 0.85 * (releaseAlpha^2); 
    
    holdZero = false;
    return;
end

holdZero     = false;
releaseAlpha = 1.0;
speedScale   = 1.0;
end

== matlab function VIRTUAL_self_driving_stack_v2/steeringCommander/MATLAB Function1 ==
  data: steerIn input; holdZero input; steerOut output; releaseAlpha input
function steerOut = smoothSteeringRelease(steerIn, holdZero, releaseAlpha)
%#codegen
    if holdZero > 0.5
        steerOut = 0.0;
    else
        % Clamp alpha for safety
        alpha = max(0.0, min(1.0, releaseAlpha));
        
        % Using alpha^4 provides a much slower initial ramp-up.
        % This prevents the 'overshoot' by ensuring the steering
        % doesn't snap to a large correction angle too early.
        steerOut = (alpha^4) * steerIn;
    end
end
